simulink model "KF_1_gdl"  (R2020b)
settings: Solver=FixedStepAuto  StartTime=0.0  StopTime=1000  FixedStep=0.02  RelTol=1e-3
values from neighbouring files (symbols this model uses):
  BARO_cov = single(1.7)/2    [init_1gdl.m]    (also in init_3_gdl_AHRS_fb.m = single(1.7)/5; init_3gdl.m; init_dati_veri.m = single(1.7)/5)
  filter_pos = tf(1,[1 1])    [init_1gdl.m]    (also in init_3_gdl_AHRS_fb.m; init_3gdl.m; init_dati_veri.m)
  GPS_cov = single([1*2, 1])/2    [init_1gdl.m]    (also in init_3_gdl_AHRS_fb.m = single([0.1*50, 0.1*50, 200*5, 200*5, 0.36])/2; init_3gdl.m = single([1*2, 1*2, 1, 1, 0.36])/2; init_dati_veri.m = single([0.1, 0.1, 200*5, 200*5, 0.36])/2)
  IMU_cov = single(15*0.07)/2    [init_1gdl.m]    (also in init_3_gdl_AHRS_fb.m = single([15*[0.07*50, 0.07*50] 15*50*0.09])/2; init_3gdl.m = single([15*[0.07, 0.07] 10*0.09])/2; init_dati_veri.m = single([15*[0.07*5, 0.07*5] 15*50*0.09])/2)
  Q = single(diag([1e-2, 1e-6, 1e-4, 1e-12]))*2    [init_1gdl.m]    (also in init_3_gdl_AHRS_fb.m = single(diag([px,vx,ax,py,vy,ay,pz,vz,az,bx,by,bz]))*2; init_3gdl.m = single(diag([px,vx,ax,py,vy,ay,pz,vz,az,bx,by,bz]))*2; init_dati_veri.m = single(diag([px,vx,ax,py,vy,ay,pz,vz,az,bx,by,bz]))*2)
  T_50 = 1/50    (= 0.02)    [init_1gdl.m]    (also in init_3_gdl_AHRS_fb.m; init_3gdl.m; init_dati_veri.m)
undefined symbols (not defined in the file or in its folder): DiscIntNeverNeededParam
libraries: cstblocks x4, simulink x2
settings Model: Creator=chiara-s  LastModifiedBy=chiara-s

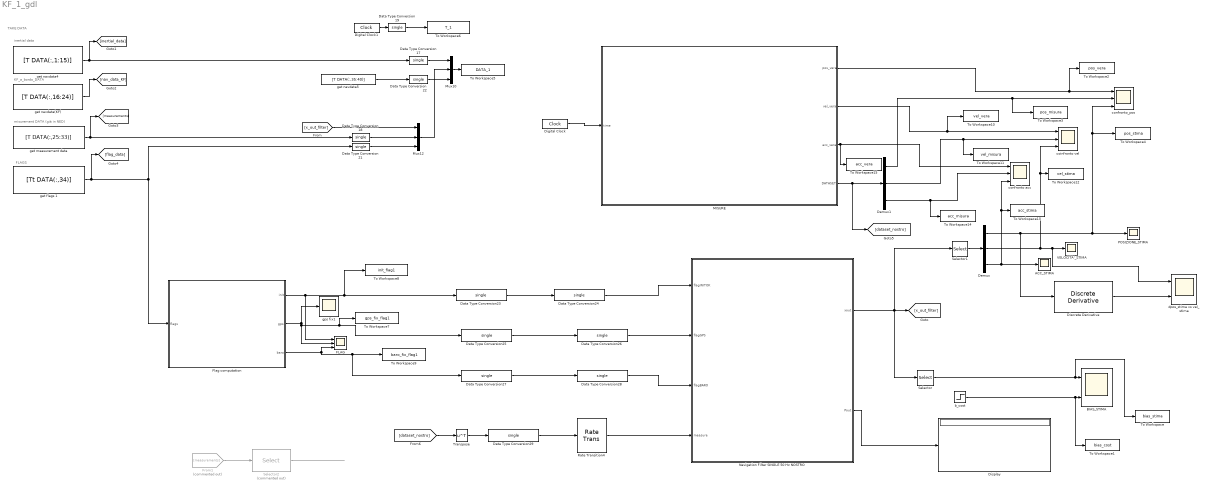
== system KF_1_gdl ==
  note: misurement DATA (già in NED)
  note: TAKE DATA
  note: inertial data
  note: KF_a_bordo_DATA
  note: FLAGS
  ACC_STIMA : Scope
  BIAS_STIMA : Scope  NumInputPorts=2
  Data Type Conversion{17..19,21..29} (12 alike) : DataTypeConversion  OutDataTypeStr=single
  Demux : Demux  Outputs=3
  Demux1 : Demux  Outputs=3
  Digital Clock : DigitalClock  SampleTime=0.02
  Digital Clock1 : DigitalClock  SampleTime=0.02
  Discrete Derivative : simulink/Discrete/Discrete Derivative  gainval=1.0  ICPrevScaledInput=0.0  OutMin=[]  OutMax=[]  OutDataType=fixdt(1, 16)  OutScaling=2^-10  DoSatur=off
  Display : Display
  FLAG : Scope  NumInputPorts=3
  Flag computation : MATLAB Function  TreatAsAtomicUnit=on
  From1 : From  Commented=on  GotoTag=measurements
  MISURE : Subsystem
  Mux10 : Mux  Inputs=3
  Mux12 : Mux  Inputs=3
  Navigation Filter SINGLE 50 Hz NOSTRO : MATLAB Function  TreatAsAtomicUnit=on  mask{Q=Q, GPS_cov=GPS_cov, IMU_cov=IMU_cov, BARO_cov=BARO_cov}
      mask prompts: Q "Q matrix"; GPS_cov "R matrix - GPS covariance [px py vx vy vz]"; IMU_cov "R matrix - IMU covariance [ax ay az]"; BARO_cov "R matrix - BARO covariance"
  POSIZIONE_STIMA : Scope
  Rate Transition4 : RateTransition  OutPortSampleTime=1/50
  Selector : Selector  InputPortWidth=4  IndexOptions=Index vector (dialog)  Indices=[4]  OutputSizes=1
  Selector1 : Selector  InputPortWidth=4  IndexOptions=Index vector (dialog)  Indices=[1 2 3]  OutputSizes=1
  Selector2 : Selector  Commented=on  InputPortWidth=9  IndexOptions=Index vector (dialog)  Indices=[1 2 3]  OutputSizes=1
  To Workspace : ToWorkspace  VariableName=bias_stima  SaveFormat=Timeseries  SampleTime=-1
  To Workspace1 : ToWorkspace  VariableName=bias_cost  SaveFormat=Timeseries  SampleTime=-1
  To Workspace10 : ToWorkspace  VariableName=vel_vera  SaveFormat=Timeseries  SampleTime=-1
  To Workspace11 : ToWorkspace  VariableName=vel_misura  SaveFormat=Timeseries  SampleTime=-1
  To Workspace12 : ToWorkspace  VariableName=vel_stima  SaveFormat=Timeseries  SampleTime=-1
  To Workspace13 : ToWorkspace  VariableName=acc_stima  SaveFormat=Timeseries  SampleTime=-1
  To Workspace14 : ToWorkspace  VariableName=acc_misura  SaveFormat=Timeseries  SampleTime=-1
  To Workspace15 : ToWorkspace  VariableName=acc_vera  SaveFormat=Timeseries  SampleTime=-1
  To Workspace2 : ToWorkspace  VariableName=pos_vera  SaveFormat=Timeseries  SampleTime=-1
  To Workspace3 : ToWorkspace  VariableName=pos_misura  SaveFormat=Timeseries  SampleTime=-1
  To Workspace4 : ToWorkspace  VariableName=pos_stima  SaveFormat=Timeseries  SampleTime=-1
  To Workspace5 : ToWorkspace  VariableName=DATA_1  SampleTime=-1
  To Workspace6 : ToWorkspace  VariableName=T_1  SampleTime=-1
  To Workspace7 : ToWorkspace  VariableName=gps_fix_flag1  SampleTime=-1
  To Workspace8 : ToWorkspace  VariableName=init_flag1  SampleTime=-1
  To Workspace9 : ToWorkspace  VariableName=baro_fix_flag1  SampleTime=-1
  Transpose : Math  Operator=transpose  SaturateOnIntegerOverflow=on
  VELOCITA'_STIMA : Scope
  b_cost : Step  Time=0  After=0.05  SampleTime=T_50
  coinfronto vel : Scope  NumInputPorts=3
  confronto acc : Scope  NumInputPorts=3
  confronto_pos : Scope  NumInputPorts=3
  dpos_stima vs vel_stima : Scope  NumInputPorts=2
  get flags 1 : FromWorkspace  VariableName=[Tt DATA(:,34)]  SampleTime=0.02  OutputAfterFinalValue=Holding final value
  "get measurement data " : FromWorkspace  VariableName=[T DATA(:,25:33)]  SampleTime=0.02  OutputAfterFinalValue=Holding final value
  get navdata(KF) : FromWorkspace  VariableName=[T DATA(:,16:24)]  SampleTime=0.02  OutputAfterFinalValue=Holding final value
  get navdata4 : FromWorkspace  VariableName=[T DATA(:,1:15)]  SampleTime=0.02  Interpolate=off  OutputAfterFinalValue=Holding final value
  get navdata5 : FromWorkspace  VariableName=[T DATA(:,35:40)]  SampleTime=0.02  Interpolate=off  OutputAfterFinalValue=Holding final value
  gps fix1 : Scope
  wires:
  Data Type Conversion19/1 -> To Workspace6/1
  Data Type Conversion25/1 -> Data Type Conversion26/1
  Data Type Conversion17/1 -> Mux10/1
  Data Type Conversion29/1 -> Rate Transition4/1
  [x_out_filter] -> Mux12/1
  Data Type Conversion28/1 -> Navigation Filter SINGLE 50 Hz NOSTRO/3(flagBARO)
  Navigation Filter SINGLE 50 Hz NOSTRO/1(xout) -> Selector/1, [x_out_filter], Selector1/1
  get navdata4/1 -> Data Type Conversion17/1, [inertial_data]
  Data Type Conversion18/1 -> Mux12/2
  Data Type Conversion24/1 -> Navigation Filter SINGLE 50 Hz NOSTRO/1(flagINITOK)
  Mux12/1 -> Mux10/2
  Data Type Conversion22/1 -> Mux10/3
  Data Type Conversion27/1 -> Data Type Conversion28/1
  Flag computation/1(init) -> FLAG/1, To Workspace8/1, Data Type Conversion23/1
  Data Type Conversion21/1 -> Mux12/3
  get navdata5/1 -> Data Type Conversion22/1
  Digital Clock1/1 -> Data Type Conversion19/1
  Navigation Filter SINGLE 50 Hz NOSTRO/2(Pout) -> Display/1
  Data Type Conversion26/1 -> Navigation Filter SINGLE 50 Hz NOSTRO/2(flagGPS)
  get flags 1/1 -> [flag_data], Flag computation/1(flags), Data Type Conversion21/1
  Rate Transition4/1 -> Navigation Filter SINGLE 50 Hz NOSTRO/4(measure)
  Data Type Conversion23/1 -> Data Type Conversion24/1
  Flag computation/2(gps) -> To Workspace7/1, Data Type Conversion25/1, FLAG/2, gps fix1/1
  "get measurement data "/1 -> [measurements], Data Type Conversion18/1
  get navdata(KF)/1 -> [nav_data_KF]
  Flag computation/3(baro) -> To Workspace9/1, Data Type Conversion27/1, FLAG/3
  Mux10/1 -> To Workspace5/1
  b_cost/1 -> To Workspace1/1, BIAS_STIMA/2
  Selector/1 -> To Workspace/1, BIAS_STIMA/1
  Selector1/1 -> Demux/1
  Demux/1 -> confronto_pos/3, To Workspace4/1, POSIZIONE_STIMA/1, Discrete Derivative/1
  Demux/2 -> To Workspace12/1, coinfronto vel/3, dpos_stima vs vel_stima/1, VELOCITA'_STIMA/1
  Demux/3 -> To Workspace13/1, confronto acc/3, ACC_STIMA/1
  MISURE/4(DATASET) -> [dataset_nostro], Demux1/1
  Digital Clock/1 -> MISURE/1(time)
  [dataset_nostro] -> Transpose/1
  Selector2/1 -> ?
  From1/1 -> Selector2/1
  Transpose/1 -> Data Type Conversion29/1
  Demux1/2 -> To Workspace11/1, coinfronto vel/2
  Demux1/3 -> To Workspace14/1, confronto acc/2
  Discrete Derivative/1 -> dpos_stima vs vel_stima/2
  MISURE/2(vel_vera) -> To Workspace10/1, coinfronto vel/1
  MISURE/3(acc_vera) -> confronto acc/1, To Workspace15/1
  MISURE/1(pos_vera) -> To Workspace2/1, confronto_pos/1
  Demux1/1 -> To Workspace3/1, confronto_pos/2

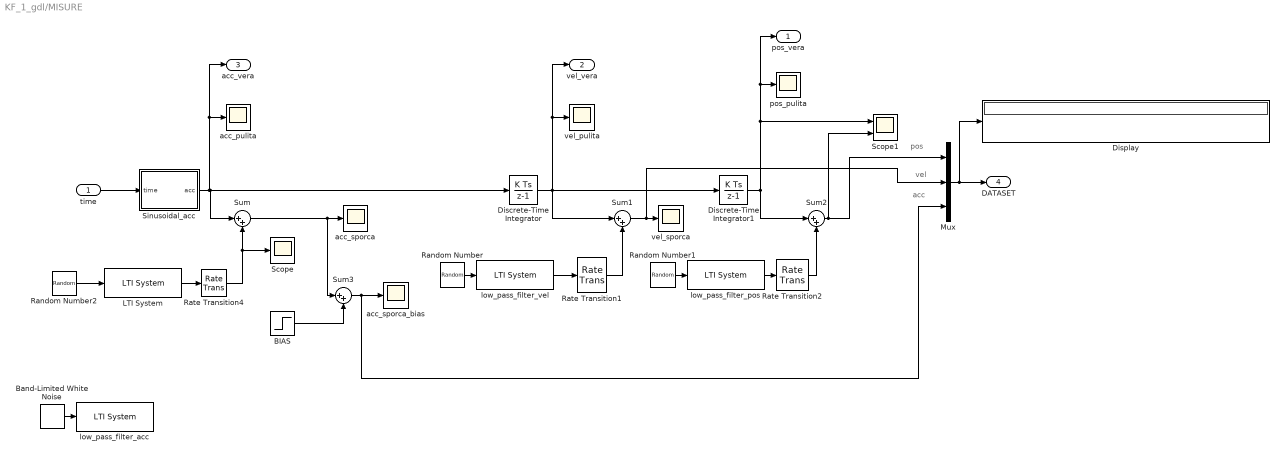
== system KF_1_gdl/MISURE ==
  note: acc
  note: vel
  note: pos
  time : Inport
  BIAS : Step  Time=0  After=0.05  SampleTime=0.02
  Band-Limited White Noise : simulink/Sources/Band-Limited White Noise  Cov=noise_gain  Ts=T_50  seed=[23341]
  Discrete-Time Integrator : DiscreteIntegrator  SampleTime=-1  ICPrevOutput=DiscIntNeverNeededParam  ICPrevScaledInput=DiscIntNeverNeededParam
  Discrete-Time Integrator1 : DiscreteIntegrator  SampleTime=-1  ICPrevOutput=DiscIntNeverNeededParam  ICPrevScaledInput=DiscIntNeverNeededParam
  Display : Display
  LTI System : cstblocks/LTI System  sys=tf(1,[0.1 1])  IC=[]
  Mux : Mux  Inputs=3
  Random Number : RandomNumber  Variance=0.16  SampleTime=0.02
  Random Number1 : RandomNumber  Seed=1  SampleTime=0.02
  Random Number2 : RandomNumber  Variance=((0.07)/2)^2  SampleTime=0.02
  Rate Transition1 : RateTransition  OutPortSampleTime=1/50
  Rate Transition2 : RateTransition  OutPortSampleTime=1/50
  Rate Transition4 : RateTransition  OutPortSampleTime=1/50
  Scope : Scope
  Scope1 : Scope  NumInputPorts=2
  Sinusoidal_acc : MATLAB Function  TreatAsAtomicUnit=on
  Sum{,1..3} (4 alike) : Sum  Inputs=|++
  acc_pulita : Scope
  acc_sporca : Scope
  acc_sporca_bias : Scope
  low_pass_filter_acc : cstblocks/LTI System  sys=filter_acc  IC=[]
  low_pass_filter_pos : cstblocks/LTI System  sys=filter_pos*10  IC=[]
  low_pass_filter_vel : cstblocks/LTI System  sys=filter_vel  IC=[]
  pos_pulita : Scope
  vel_pulita : Scope
  vel_sporca : Scope
  pos_vera : Outport
  vel_vera : Outport  Port=2
  acc_vera : Outport  Port=3
  DATASET : Outport  Port=4
  wires:
  Sinusoidal_acc/1(acc) -> acc_vera/1, acc_pulita/1, Sum/1, Discrete-Time Integrator/1
  Mux/1 -> Display/1, DATASET/1
  Discrete-Time Integrator/1 -> Sum1/1, Discrete-Time Integrator1/1, vel_pulita/1, vel_vera/1
  time/1 -> Sinusoidal_acc/1(time)
  Discrete-Time Integrator1/1 -> Sum2/1, pos_vera/1, pos_pulita/1, Scope1/1
  Sum/1 -> Sum3/1, acc_sporca/1
  LTI System/1 -> Rate Transition4/1
  low_pass_filter_vel/1 -> Rate Transition1/1
  Sum1/1 -> Mux/2, vel_sporca/1
  Sum2/1 -> Scope1/2, Mux/1
  Random Number/1 -> low_pass_filter_vel/1
  Random Number1/1 -> low_pass_filter_pos/1
  BIAS/1 -> Sum3/2
  Sum3/1 -> acc_sporca_bias/1, Mux/3
  Rate Transition1/1 -> Sum1/2
  low_pass_filter_pos/1 -> Rate Transition2/1
  Rate Transition2/1 -> Sum2/2
  Random Number2/1 -> LTI System/1
  Rate Transition4/1 -> Scope/1, Sum/2
  Band-Limited White Noise/1 -> low_pass_filter_acc/1

== matlab function KF_1_gdl/MISURE/Sinusoidal_acc ==
  settings: updateMethod=DISCRETE  sampleTime=0.02
  data: time input; acc output
function acc = fcn(time)

t = time;

a = 0.02*sin(0.01*t);
b = (0.03)*sin(0.05*t + pi);
c = (0.04)*sin(0.03*t + pi/2);
if t >= 0 && t < 107 
    acc = 0;
else
    acc = a + b + c;
    acc = acc - 0.0018;
end

end

== matlab function KF_1_gdl/Flag computation ==
  data: flags input; init output; gps output; baro output
function [init,gps,baro] = fcn(flags)
%#codegen
%flags = init*100 + baro*10 + gps;

% centinaia: 
if flags > 50
    init = 1;
else
    init = 0;
end
%decine 
if flags-init*100 > 5
    baro = 1;
else
    baro = 0;
end
%unità
if flags-init*100-baro*10 > 0.5
    gps = 1;
else
    gps = 0;
end


% flags = 100 + 10 + 1;
% init 100
% init + gps 110
% init + gps + baro = 111
% init + baro = 101

== matlab function KF_1_gdl/Navigation Filter SINGLE 50 Hz NOSTRO ==
  data: flagINITOK input single size=1; flagGPS input single size=1; flagBARO input single size=1; xout output single size=4; measure input single size=3; Q parameter single size=[4,4]; GPS_cov parameter single size=2; BARO_cov parameter single size=1; IMU_cov parameter single size=1; Pout output single
function [xout,Pout] = GPS_BARO_KF_opt( flagINITOK, flagGPS, flagBARO, measure, Q, GPS_cov, BARO_cov, IMU_cov)

%% definition of variables
persistent P %covariance matrix 
persistent x %state vector
persistent filter_running
%filter matrices and constants
persistent A B 
persistent C_GPS_tot R_GPS_tot C_GPS_pos_vel R_GPS_pos_vel C_BARO R_BARO C_IMU R_IMU

if isempty(P)
   % esce qualcosa
     P = single(1)*eye(4); % Q da cambiare (dimensioni e valori)
%      P(3,3) = 50;
     %P(2,2) = 0.5; 
     P(4,4) = 50; 



    % Augmented State (pos, vel, acc, bias  -  1 gdl)
    x = single(zeros(4,1));
    
    filter_running = logical(false); %filter starts in OFF, must wait for flagINITOK to become true
    
    dt = single(0.02); 
    %u  = 0;
    A =    [1, dt,  0.5*dt^2, 0;
            0,  1,        dt, 0;
            0,  0,         1, 0;
            0,  0,         0, 1];
        

    
    % Augmented B
    B = single(eye(4,1));

    % Augmented Covariance state matrix (eps = bias accelerometer - body frame)
    % p|v|a|eps|
    % Q from init 

    % Covariance output matrix
    % GPS covariances = p|v|
    % GPS_cov  = [0.03, 0.05, 0.016, 0.014, 0.36]; from init
    % IMU covariances = a
    % IMU_cov  = 1000*[0.07, 0.07, 0.09];    from init
    % BARO_cov =  1.7; from init 

% Rotation Matrix from body to navigation frame
%     phi = euler_in(1);
%     theta = euler_in(2);
%     psi = euler_in(3);
%     C = rotation(phi,theta,psi);
    
    %output matrices 
    %tutte le misure disponibili 
    C_GPS_tot = single([ 1  0  0  0;
                         0  1  0  0;
                         0  0  1  1]);
                                                                                                                                                                                                                                                                                                                                                                                                                                                                                                                                                                                                                                                                                                                                                                                                                                     ;
    R_GPS_tot = single(diag([GPS_cov(1),GPS_cov(2), IMU_cov]));
    
    % vel GPS, pos GPS & IMU
    C_GPS_pos_vel =  single([ 1  0  0  0;
                              0  1  0  0;
                              0  0  1  1]);
                         
    R_GPS_pos_vel = single(diag([GPS_cov(1),GPS_cov(2), IMU_cov]));
    
    % Baro & IMU
    C_BARO = single([ 1  0  0  0;
                      0  0  1  1]);
                 
    R_BARO = single(diag([BARO_cov, IMU_cov]));
    R_BARO = R_BARO*2;
                 
    % solo IMU
    C_IMU = single([0, 0, 1, 1]);
                
    R_IMU = single(IMU_cov);
    
end


% x 4x1
%% initialization 
if and(not(filter_running),flagINITOK),
    % if filter is not running and initialization can be performed 
    % => initialize state = measure
    % => notify filter is running
    x= [measure; 0];
    filter_running = true;
end


%% TODO: capire che senso ha mettere u = 0 sempre 
u  = single(0);


if filter_running, 
    %% select update type (removed fuse types with separate gps pos and vel flags)
    if(flagGPS && flagBARO)
        fuse = 1;
    elseif(flagGPS)
        fuse = 2;
    elseif(flagBARO)
        fuse = 7;
    else
        fuse = 8;
    end

    %% Prediction
    [x, P] = predict(A, B, x, u, Q, P);


    %% Update
    switch fuse
        case 1
            % all measurements
            y = [measure(1), measure(2), measure(3)]';
            [x, P] = update(A, C_GPS_tot, x, y, P, R_GPS_tot);
        case 2
            % measurements of: pos GPS, vel GPS, IMU
            y = [measure(1), measure(2), measure(3)]';
            [x, P] = update(A, C_GPS_pos_vel, x, y, P, R_GPS_pos_vel);
        case 7
            % measurements of: BARO, IMU
            y = [measure(1), measure(3)]';
            [x, P] = update(A, C_BARO, x, y, P, R_BARO);
        case 8
            y = [measure(3)]';
            [x, P] = update(A, C_IMU, x, y, P, R_IMU);
    end
end

xout = x;
Pout = P;
end

function [x, P] = predict(A, B, x, u, Q, P)
    x = A*x + B*u;
    P = A*P*A' + Q;
end

function [x, P] = update(A, C, x, y, P, R)
    K = P*C'*inv(R + C*P*C');       % al max 4x3 se tutti sensori attivi
    x = x + K*(y - C*x);
    P = (eye(4) - K*C)*P;
    %P = 0.5*(P + transpose(P)); secondo me ci va, non dovrebbe fare male
end
